simulink model "regulatory"  (R2016b)
settings: Solver=FixedStepAuto  StartTime=0.0  StopTime=15  FixedStep=0.001  RelTol=1e-3  EnableMultiTasking=on
libraries: simulink x1
settings Model: Creator=student  LastModifiedBy=lenovo
settings OptimizationCC: LifeSpan=inf
settings DebuggingCC: SFUnexpectedBacktrackingDiag=warning  SFNoUnconditionalDefaultTransitionDiag=warning  SFExecutionAtInitializationDiag=none
settings GRTTargetCC: TargetLangStandard=C89/C90 (ANSI)  GeneratePreprocessorConditionals=Disable all
settings ConfigComp: CovMetricSettings=dw  CovHtmlReporting=on  CovSaveCumulativeToWorkspaceVar=on  CovSaveSingleToWorkspaceVar=on  CovExternalEMLEnable=off

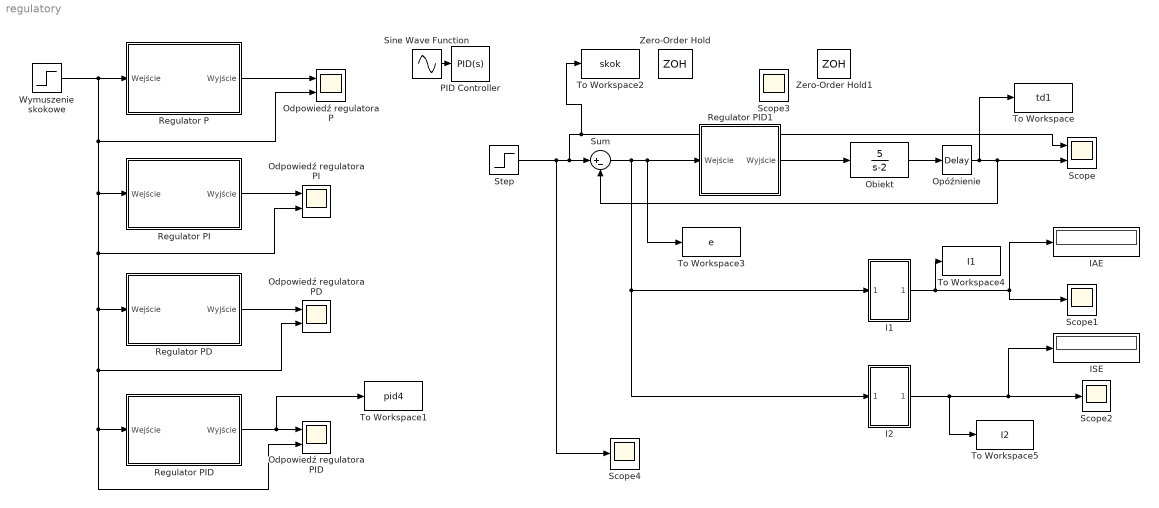
== system regulatory ==
  I1 : Subsystem
  I2 : Subsystem
  IAE : Display
  ISE : Display
  Obiekt : TransferFcn  Numerator=[5]  Denominator=[1 -2]
  Odpowiedź regulatora P : Scope  NumInputPorts=2
  Odpowiedź regulatora PID : Scope  NumInputPorts=2
  Odpowiedź regulatoraPD : Scope  NumInputPorts=2
  Odpowiedź regulatoraPI : Scope  NumInputPorts=2
  Opóźnienie : TransportDelay  DelayTime=0.01
  PID Controller : simulink/Continuous/PID Controller  Controller=PID  TimeDomain=Continuous-time  SampleTime=-1  IntegratorMethod=Forward Euler  FilterMethod=Forward Euler  Form=Parallel  UseFilter=on  ControllerParametersSource=internal  P=4.14938706550423  I=8.45365813879702  D=0.0164166995342469  N=37.0867704416697  InitialConditionSource=internal  InitialConditionForIntegrator=0  InitialConditionForFilter=0  ExternalReset=none  LimitOutput=off  UpperSaturationLimit=inf  LowerSaturationLimit=-inf  LinearizeAsGain=on  AntiWindupMode=none  Kb=1  TrackingMode=off  Kt=1  PParamMin=[]  PParamMax=[]  IParamMin=[]  IParamMax=[]  DParamMin=[]  DParamMax=[]  NParamMin=[]  NParamMax=[]  KbParamMin=[]  KbParamMax=[]  KtParamMin=[]  KtParamMax=[]  POutMin=[]  POutMax=[]  IOutMin=[]  IOutMax=[]  DOutMin=[]  DOutMax=[]  NOutMin=[]  NOutMax=[]  KbOutMin=[]  KbOutMax=[]  KtOutMin=[]  KtOutMax=[]  IntegratorOutMin=[]  IntegratorOutMax=[]  FilterOutMin=[]  FilterOutMax=[]  SumOutMin=[]  SumOutMax=[]  SumI1OutMin=[]  SumI1OutMax=[]  SumI2OutMin=[]  SumI2OutMax=[]  SumI3OutMin=[]  SumI3OutMax=[]  SumDOutMin=[]  SumDOutMax=[]  SaturationOutMin=[]  SaturationOutMax=[]  IntegratorContinuousStateAttributes=''  IntegratorStateMustResolveToSignalObject=off  IntegratorRTWStateStorageClass=Auto  FilterContinuousStateAttributes=''  FilterStateMustResolveToSignalObject=off  FilterRTWStateStorageClass=Auto  DifferentiatorICPrevScaledInput=0  DifferentiatorOutMin=[]  DifferentiatorOutMax=[]
  Regulator P : Subsystem  mask{kp=10, Ti=0, Td=0, T=0}
  Regulator PD : Subsystem  mask{kp=3, Ti=0, Td=0.5, T=1}
  Regulator PI : Subsystem  mask{kp=5, Ti=5, Td=0, T=0}
  Regulator PID : Subsystem  mask{kp=3, Ti=4, Td=8, T=2}
  Regulator PID1 : Subsystem  mask{kp=5, Ti=1, Td=0, T=0.04}
  Scope : Scope  NumInputPorts=2
  Scope1 : Scope
  Scope2 : Scope
  Scope3 : Scope  NumInputPorts=2
  Scope4 : Scope
  Sine Wave Function : Sin  Frequency=3  SampleTime=0
  Step : Step  SampleTime=0
  Sum : Sum  Inputs=|+-
  To Workspace : ToWorkspace  VariableName=td1  SaveFormat=Timeseries  SampleTime=-1
  To Workspace1 : ToWorkspace  VariableName=pid4  SaveFormat=Timeseries  SampleTime=-1
  To Workspace2 : ToWorkspace  VariableName=skok  SaveFormat=Timeseries  SampleTime=-1
  To Workspace3 : ToWorkspace  VariableName=e  SaveFormat=Timeseries  SampleTime=-1
  To Workspace4 : ToWorkspace  VariableName=I1  SaveFormat=Timeseries  SampleTime=-1
  To Workspace5 : ToWorkspace  VariableName=I2  SaveFormat=Timeseries  SampleTime=-1
  Wymuszenie skokowe : Step  SampleTime=0
  Zero-Order Hold : ZeroOrderHold  SampleTime=0.01
  Zero-Order Hold1 : ZeroOrderHold  SampleTime=0.01
  wires:
  Wymuszenie skokowe/1 -> Odpowiedź regulatora P/2, Regulator PI/1(Wejście), Odpowiedź regulatoraPI/2, Regulator PD/1(Wejście), Odpowiedź regulatoraPD/2, Odpowiedź regulatora PID/2, Regulator PID/1(Wejście), Regulator P/1(Wejście)
  Regulator P/1(Wyjście) -> Odpowiedź regulatora P/1
  Regulator PI/1(Wyjście) -> Odpowiedź regulatoraPI/1
  Regulator PD/1(Wyjście) -> Odpowiedź regulatoraPD/1
  Regulator PID/1(Wyjście) -> To Workspace1/1, Odpowiedź regulatora PID/1
  Obiekt/1 -> Opóźnienie/1
  Opóźnienie/1 -> To Workspace/1, Sum/2, Scope/2
  I1/1(Out1) -> To Workspace4/1, IAE/1, Scope1/1
  I2/1(Out1) -> To Workspace5/1, ISE/1, Scope2/1
  Sum/1 -> Regulator PID1/1(Wejście), To Workspace3/1, I2/1(In1), I1/1(In1)
  Step/1 -> Scope4/1, To Workspace2/1, Scope/1, Sum/1
  Regulator PID1/1(Wyjście) -> Obiekt/1
  Sine Wave Function/1 -> PID Controller/1

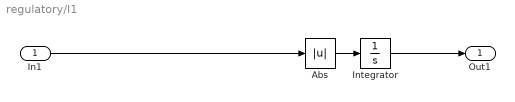
== system regulatory/I1 ==
  In1 : Inport
  Abs : Abs
  Integrator : Integrator
  Out1 : Outport
  wires:
  Integrator/1 -> Out1/1
  Abs/1 -> Integrator/1
  In1/1 -> Abs/1

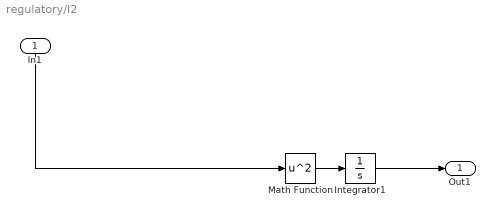
== system regulatory/I2 ==
  In1 : Inport
  Integrator1 : Integrator
  Math Function : Math  Operator=square  SaturateOnIntegerOverflow=on
  Out1 : Outport
  wires:
  Math Function/1 -> Integrator1/1
  Integrator1/1 -> Out1/1
  In1/1 -> Math Function/1

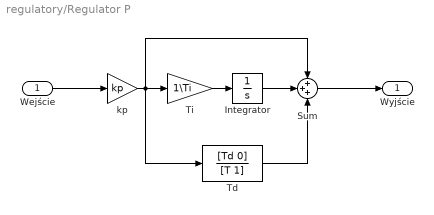
== system regulatory/Regulator P ==
  Wejście : Inport
  Integrator : Integrator
  Sum : Sum  Inputs=+++
  Td : TransferFcn  Numerator=[Td 0]  Denominator=[T 1]
  Ti : Gain  Gain=1\Ti
  kp : Gain  Gain=kp
  Wyjście : Outport
  wires:
  Sum/1 -> Wyjście/1
  Wejście/1 -> kp/1
  Ti/1 -> Integrator/1
  kp/1 -> Td/1, Sum/1, Ti/1
  Integrator/1 -> Sum/2
  Td/1 -> Sum/3

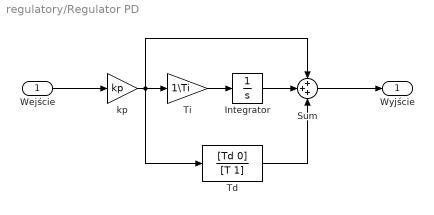
== system regulatory/Regulator PD ==
  Wejście : Inport
  Integrator : Integrator
  Sum : Sum  Inputs=+++
  Td : TransferFcn  Numerator=[Td 0]  Denominator=[T 1]
  Ti : Gain  Gain=1\Ti
  kp : Gain  Gain=kp
  Wyjście : Outport
  wires:
  Sum/1 -> Wyjście/1
  Wejście/1 -> kp/1
  Ti/1 -> Integrator/1
  kp/1 -> Td/1, Sum/1, Ti/1
  Integrator/1 -> Sum/2
  Td/1 -> Sum/3

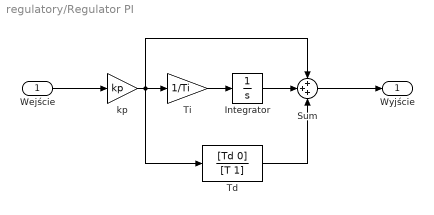
== system regulatory/Regulator PI ==
  Wejście : Inport
  Integrator : Integrator
  Sum : Sum  Inputs=+++
  Td : TransferFcn  Numerator=[Td 0]  Denominator=[T 1]
  Ti : Gain  Gain=1/Ti
  kp : Gain  Gain=kp
  Wyjście : Outport
  wires:
  Sum/1 -> Wyjście/1
  Wejście/1 -> kp/1
  Ti/1 -> Integrator/1
  kp/1 -> Td/1, Sum/1, Ti/1
  Integrator/1 -> Sum/2
  Td/1 -> Sum/3

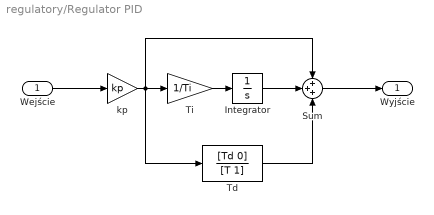
== system regulatory/Regulator PID ==
  Wejście : Inport
  Integrator : Integrator
  Sum : Sum  Inputs=+++
  Td : TransferFcn  Numerator=[Td 0]  Denominator=[T 1]
  Ti : Gain  Gain=1/Ti
  kp : Gain  Gain=kp
  Wyjście : Outport
  wires:
  Sum/1 -> Wyjście/1
  Wejście/1 -> kp/1
  Ti/1 -> Integrator/1
  kp/1 -> Td/1, Sum/1, Ti/1
  Integrator/1 -> Sum/2
  Td/1 -> Sum/3

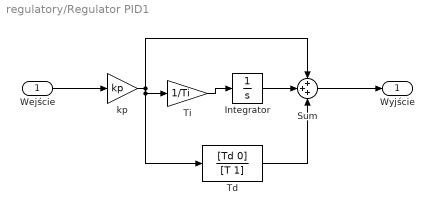
== system regulatory/Regulator PID1 ==
  Wejście : Inport
  Integrator : Integrator
  Sum : Sum  Inputs=+++
  Td : TransferFcn  Numerator=[Td 0]  Denominator=[T 1]
  Ti : Gain  Gain=1/Ti
  kp : Gain  Gain=kp
  Wyjście : Outport
  wires:
  Sum/1 -> Wyjście/1
  Wejście/1 -> kp/1
  Ti/1 -> Integrator/1
  kp/1 -> Td/1, Ti/1, Sum/1
  Integrator/1 -> Sum/2
  Td/1 -> Sum/3
